simulink model "RefModel_Navfilter"  (R2020b)
settings: Solver=ode1  StartTime=0.0  StopTime=inf  FixedStep=Ts_Navi.Ts_Base  RelTol=1e-3
values from neighbouring files (symbols this model uses):
  NAVI_PARAM_V10 = INIT_Navi_V10(NaviSimParam.Ts_Base)    [SetAlgoParam_Navi.m]
  NAVI_PARAM_V1000 = INIT_Navi_V1000(NaviSimParam.Ts_Base)    [SetAlgoParam_Navi.m]
undefined symbols (not defined in the file or in its folder): ENUM_SensorHealthStatus, NAVI_PARAM_BASE
libraries: aerolibobsolete x1
(part 1 of 2)
settings Model: PauseTimes=[308,310,12]  Creator=sl  LastModifiedBy=sl
settings DataIOCC: SaveOutput=off  SaveTime=off
settings OptimizationCC: DefaultParameterBehavior=Inlined  EnhancedBackFolding=on  PassReuseOutputArgsAs=Individual arguments  ZeroExternalMemoryAtStartup=off  ZeroInternalMemoryAtStartup=off  OptimizeBlockOrder=speed  DifferentSizesBufferReuse=on  OptimizationCustomize=off  EfficientTunableParamExpr=on
settings DebuggingCC: InheritedTsInSrcMsg=none  ParameterPrecisionLossMsg=none  ParameterTunabilityLossMsg=error  UnconnectedInputMsg=none  UnconnectedOutputMsg=none  UnconnectedLineMsg=none  SFUnusedDataAndEventsDiag=none
settings HardwareCC: ProdBitPerPointer=32  ProdBitPerSizeT=32  ProdBitPerPtrDiffT=32  ProdLargestAtomicInteger=Long  ProdLargestAtomicFloat=Double  ProdWordSize=32  ProdHWDeviceType=ARM Compatible->ARM Cortex
settings ModelReferenceCC: ModelReferenceNumInstancesAllowed=Single
settings SFSimCC: MATLABDynamicMemAlloc=off
settings RTWCC: Description=Embedded Coder  SystemTargetFile=ert.tlc  TemplateMakefile=ert_default_tmf  GenerateReport=on  IncludeHyperlinkInReport=on  LaunchReport=on  GenerateTraceInfo=on  GenerateTraceReport=on  GenerateTraceReportSl=on  GenerateTraceReportSf=on  GenerateTraceReportEml=on
settings CodeAppCC: ForceParamTrailComments=on  IgnoreCustomStorageClasses=off  MaxIdLength=48  OperatorAnnotations=on  SimulinkDataObjDesc=on  SFDataObjDesc=on  InsertBlockDesc=on
settings ERTTargetCC: TargetLangStandard=C99 (ISO)  GenerateSampleERTMain=on  CombineOutputUpdateFcns=off  LogVarNameModifier=none  SupportVariableSizeSignals=on  InlinedParameterPlacement=NonHierarchical  ERTCustomFileTemplate=example_file_process.tlc

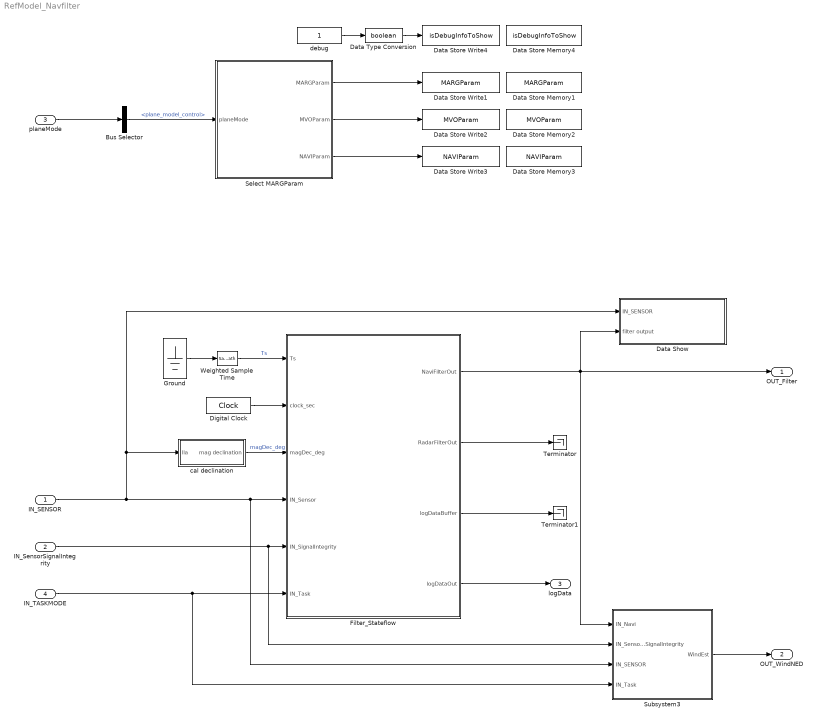
== system RefModel_Navfilter ==
  IN_SENSOR : Inport  OutDataTypeStr=Bus: BUS_SENSOR  BusOutputAsStruct=on
  IN_SensorSignalIntegrity : Inport  Port=2  OutDataTypeStr=Bus: BUS_NAVI_SensorSignalIntegrity  BusOutputAsStruct=on
  planeMode : Inport  Port=3  OutDataTypeStr=Bus: BUS_SYSTEMINFO_INPUT
  IN_TASKMODE : Inport  Port=4  OutDataTypeStr=Bus: BUS_TASK_PATH_OutParam  BusOutputAsStruct=on
  Bus Selector : BusSelector  OutputSignals=plane_model_control
  Data Show : Subsystem
  Data Store Memory1 : DataStoreMemory  DataStoreName=MARGParam  ReadBeforeWriteMsg=warning  WriteAfterWriteMsg=warning  WriteAfterReadMsg=warning  ShowAdditionalParam=off  OutDataTypeStr=Bus: BUS_NAVIPARAM_MARG  Dimensions=1
  Data Store Memory2 : DataStoreMemory  DataStoreName=MVOParam  ReadBeforeWriteMsg=warning  WriteAfterWriteMsg=warning  WriteAfterReadMsg=warning  ShowAdditionalParam=off  OutDataTypeStr=Bus: BUS_NAVIPARAM_MVO  Dimensions=1
  Data Store Memory3 : DataStoreMemory  DataStoreName=NAVIParam  ReadBeforeWriteMsg=warning  WriteAfterWriteMsg=warning  WriteAfterReadMsg=warning  ShowAdditionalParam=off  OutDataTypeStr=Bus: BUS_NAVIPARAM  Dimensions=1
  Data Store Memory4 : DataStoreMemory  DataStoreName=isDebugInfoToShow  ReadBeforeWriteMsg=warning  WriteAfterWriteMsg=warning  WriteAfterReadMsg=warning  ShowAdditionalParam=off  OutDataTypeStr=boolean  Dimensions=1
  Data Store Write1 : DataStoreWrite  DataStoreName=MARGParam
  Data Store Write2 : DataStoreWrite  DataStoreName=MVOParam
  Data Store Write3 : DataStoreWrite  DataStoreName=NAVIParam
  Data Store Write4 : DataStoreWrite  DataStoreName=isDebugInfoToShow
  Data Type Conversion : DataTypeConversion  OutDataTypeStr=boolean
  Digital Clock : DigitalClock  SampleTime=-1
  Filter_Stateflow : Stateflow chart  TreatAsAtomicUnit=on
      settings: PortSchema="{\"entries\":[{\"content\":{\"sides\":[{\"content\":{\"connectorIds\":[\"In1\",\"In2\",\"In3\",\"In4\",\"In5\",\"In6\"]},\"type\":\"ConnectorPlacement.EquallySpacedRectSide\",\"uuid\":\"09dead05-b0d6-46e3-b4df-7e330e053911\"},{\"content\":{\"connectorIds\":[\"Out2\",\"Out1\",\"Out3\",\"Out4\"],\"side\":\"RIGHT\"},\"type\":\"ConnectorPlacement.EquallySpacedRectSide\",\"uuid\":\"42007dbc-3269-4462-8f8b-2c35f13a3107\"},{\"content\":{\"connectorIds\":[],\"side\":\"TOP\"},\"type\":\"ConnectorPlacement.EquallySpacedRectSide\",\"uuid\":\"e6ce5443-da4b-4773-901c-23b39c5492a3\"}]},\"type\":\"ConnectorPlacement.EquallySpacedConnector\",\"uuid\":\"f5fda4a3-ef90-4dff-b16b-01a3b267f071\"}],\"packageUris\":[\"http://schema.mathworks.com/mf0/Connector/R2020b\"],\"version\":\"1.0\"}"
  Ground : Ground
  Select MARGParam : Subsystem
  Subsystem3 : Subsystem
  Terminator : Terminator
  Terminator1 : Terminator
  Weighted Sample Time : SampleTimeMath  TsampMathOp=Ts Only
  cal declination : Subsystem
  debug : Constant
  OUT_Filter : Outport  OutDataTypeStr=Bus: BUS_NAVI_FilterOut  BusOutputAsStruct=on
  OUT_WindNED : Outport  Port=2  OutDataTypeStr=Bus: BUS_NAVI_GlobalWindEst  BusOutputAsStruct=on
  logData : Outport  Port=3  OutDataTypeStr=Bus: BUS_NAVI_SingleLog  BusOutputAsStruct=on
  wires:
  IN_SensorSignalIntegrity/1 -> Subsystem3/2(IN_SensorSignalIntegrity), Filter_Stateflow/5(IN_SignalIntegrity)
  IN_SENSOR/1 -> cal declination/1(lla), Data Show/1(IN_SENSOR), Subsystem3/3(IN_SENSOR), Filter_Stateflow/4(IN_Sensor)
  Digital Clock/1 -> Filter_Stateflow/2(clock_sec)
  Weighted Sample Time/1 -> Filter_Stateflow/1(Ts)  "Ts"
  Ground/1 -> Weighted Sample Time/1
  Subsystem3/1(WindEst) -> OUT_WindNED/1
  Select MARGParam/1(MARGParam) -> Data Store Write1/1
  planeMode/1 -> Bus Selector/1
  Bus Selector/1 -> Select MARGParam/1(planeMode)  "<plane_model_control>"
  Select MARGParam/2(MVOParam) -> Data Store Write2/1
  Select MARGParam/3(NAVIParam) -> Data Store Write3/1
  IN_TASKMODE/1 -> Subsystem3/4(IN_Task), Filter_Stateflow/6(IN_Task)
  cal declination/1(mag declination) -> Filter_Stateflow/3(magDec_deg)  "magDec_deg"
  Data Type Conversion/1 -> Data Store Write4/1
  debug/1 -> Data Type Conversion/1
  Filter_Stateflow/4(logDataOut) -> logData/1
  Filter_Stateflow/2(NaviFilterOut) -> Subsystem3/1(IN_Navi), OUT_Filter/1, Data Show/2(filter output)
  Filter_Stateflow/1(RadarFilterOut) -> Terminator/1
  Filter_Stateflow/3(logDataBuffer) -> Terminator1/1

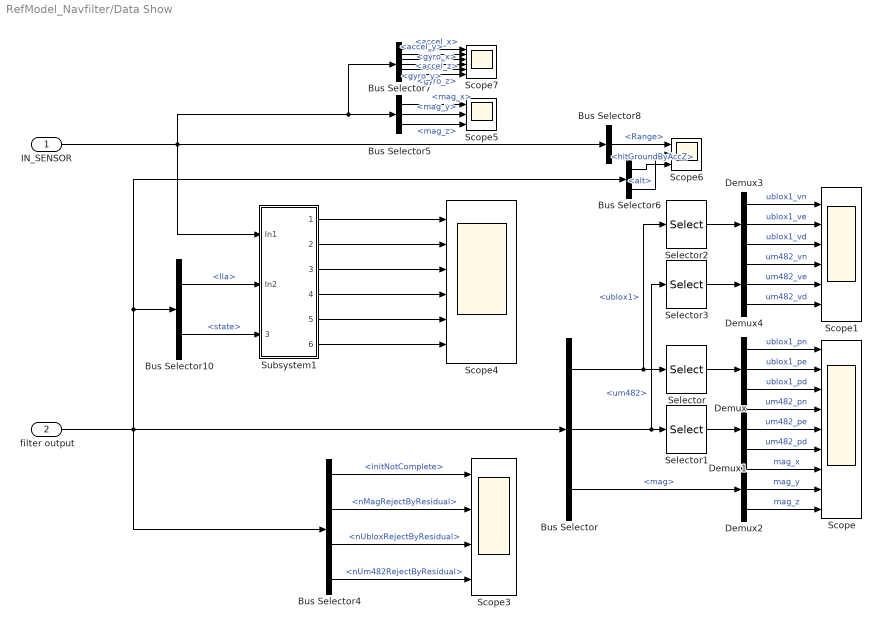
== system RefModel_Navfilter/Data Show ==
  IN_SENSOR : Inport
  filter output : Inport  Port=2
  Bus Selector : BusSelector  OutputSignals=innovMARG.ublox1,innovMARG.um482,innovMARG.mag
  Bus Selector10 : BusSelector  OutputSignals=lla,state
  Bus Selector4 : BusSelector  OutputSignals=Status.initNotComplete,Status.nMagRejectByResidual,Status.nUbloxRejectByResidual,Status.nUm482RejectByResidual
  Bus Selector5 : BusSelector  OutputSignals=mag2.mag_x,mag2.mag_y,mag2.mag_z
  Bus Selector6 : BusSelector  OutputSignals=hitGroundByAccZ,alt
  Bus Selector7 : BusSelector  OutputSignals=IMU1.accel_x,IMU1.accel_y,IMU1.accel_z,IMU1.gyro_x,IMU1.gyro_y,IMU1.gyro_z
  Bus Selector8 : BusSelector  OutputSignals=radar1.Range
  Demux{,1..4} (5 alike) : Demux  Outputs=3
  Scope : Scope  NumInputPorts=9
  Scope1 : Scope  NumInputPorts=6
  Scope3 : Scope  NumInputPorts=4
  Scope4 : Scope  NumInputPorts=6
  Scope5 : Scope  NumInputPorts=3
  Scope6 : Scope  NumInputPorts=3
  Scope7 : Scope  NumInputPorts=6
  Selector : Selector  InputPortWidth=6  IndexOptions=Index vector (dialog)  Indices=[1:3]  OutputSizes=1
  Selector1 : Selector  InputPortWidth=6  IndexOptions=Index vector (dialog)  Indices=[1:3]  OutputSizes=1
  Selector2 : Selector  InputPortWidth=6  IndexOptions=Index vector (dialog)  Indices=[4:6]  OutputSizes=1
  Selector3 : Selector  InputPortWidth=6  IndexOptions=Index vector (dialog)  Indices=[4:6]  OutputSizes=1
  Subsystem1 : Subsystem
  wires:
  Demux/3 -> Scope/3  "ublox1_pd"
  Subsystem1/5(Out5) -> Scope4/5
  IN_SENSOR/1 -> Subsystem1/1(In1), Bus Selector7/1, Bus Selector5/1, Bus Selector8/1
  Bus Selector10/2 -> Subsystem1/3(stateEst)  "<state>"
  Demux2/1 -> Scope/7  "mag_x"
  Bus Selector10/1 -> Subsystem1/2(In2)  "<lla>"
  Subsystem1/6(Out6) -> Scope4/6
  Demux2/2 -> Scope/8  "mag_y"
  Bus Selector5/3 -> Scope5/3  "<mag_z>"
  Demux1/1 -> Scope/4  "um482_pn"
  Selector3/1 -> Demux4/1
  Demux/2 -> Scope/2  "ublox1_pe"
  Demux3/3 -> Scope1/3  "ublox1_vd"
  Bus Selector7/4 -> Scope7/4  "<gyro_x>"
  Bus Selector/2 -> Selector3/1, Selector1/1  "<um482>"
  Bus Selector7/6 -> Scope7/6  "<gyro_z>"
  Bus Selector/1 -> Selector2/1, Selector/1  "<ublox1>"
  Demux1/3 -> Scope/6  "um482_pd"
  Selector/1 -> Demux/1
  Bus Selector7/5 -> Scope7/5  "<gyro_y>"
  Bus Selector5/1 -> Scope5/1  "<mag_x>"
  Demux4/1 -> Scope1/4  "um482_vn"
  Demux4/2 -> Scope1/5  "um482_ve"
  Demux/1 -> Scope/1  "ublox1_pn"
  Bus Selector7/1 -> Scope7/1  "<accel_x>"
  Bus Selector/3 -> Demux2/1  "<mag>"
  Demux4/3 -> Scope1/6  "um482_vd"
  Demux3/2 -> Scope1/2  "ublox1_ve"
  Selector2/1 -> Demux3/1
  Bus Selector7/3 -> Scope7/3  "<accel_z>"
  Subsystem1/4(Out4) -> Scope4/4
  Demux1/2 -> Scope/5  "um482_pe"
  Subsystem1/1(Out1) -> Scope4/1
  Demux3/1 -> Scope1/1  "ublox1_vn"
  Demux2/3 -> Scope/9  "mag_z"
  Bus Selector5/2 -> Scope5/2  "<mag_y>"
  Subsystem1/2(Out2) -> Scope4/2
  Bus Selector6/1 -> Scope6/3  "<hitGroundByAccZ>"
  Bus Selector7/2 -> Scope7/2  "<accel_y>"
  Bus Selector6/2 -> Scope6/2  "<alt>"
  Subsystem1/3(Out3) -> Scope4/3
  Bus Selector8/1 -> Scope6/1  "<Range>"
  Selector1/1 -> Demux1/1
  Bus Selector4/2 -> Scope3/2  "<nMagRejectByResidual>"
  Bus Selector4/1 -> Scope3/1  "<initNotComplete>"
  Bus Selector4/4 -> Scope3/4  "<nUm482RejectByResidual>"
  Bus Selector4/3 -> Scope3/3  "<nUbloxRejectByResidual>"
  filter output/1 -> Bus Selector4/1, Bus Selector/1, Bus Selector6/1, Bus Selector10/1

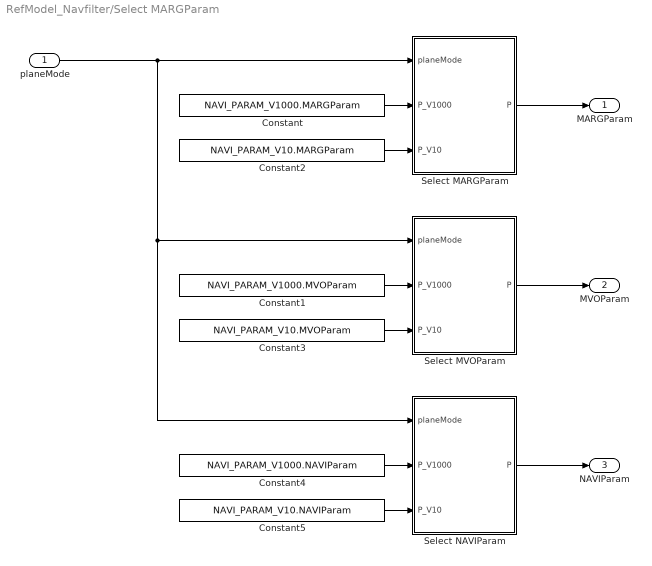
== system RefModel_Navfilter/Select MARGParam ==
  planeMode : Inport
  Constant : Constant  Value=NAVI_PARAM_V1000.MARGParam  OutDataTypeStr=Bus: BUS_NAVIPARAM_MARG
  Constant1 : Constant  Value=NAVI_PARAM_V1000.MVOParam  OutDataTypeStr=Bus: BUS_NAVIPARAM_MVO
  Constant2 : Constant  Value=NAVI_PARAM_V10.MARGParam  OutDataTypeStr=Bus: BUS_NAVIPARAM_MARG
  Constant3 : Constant  Value=NAVI_PARAM_V10.MVOParam  OutDataTypeStr=Bus: BUS_NAVIPARAM_MVO
  Constant4 : Constant  Value=NAVI_PARAM_V1000.NAVIParam  OutDataTypeStr=Bus: BUS_NAVIPARAM
  Constant5 : Constant  Value=NAVI_PARAM_V10.NAVIParam  OutDataTypeStr=Bus: BUS_NAVIPARAM
  Select MARGParam : MATLAB Function  TreatAsAtomicUnit=on
  Select MVOParam : MATLAB Function  TreatAsAtomicUnit=on
  Select NAVIParam : MATLAB Function  TreatAsAtomicUnit=on
  MARGParam : Outport
  MVOParam : Outport  Port=2
  NAVIParam : Outport  Port=3
  wires:
  Constant/1 -> Select MARGParam/2(P_V1000)
  Constant2/1 -> Select MARGParam/3(P_V10)
  Select MARGParam/1(P) -> MARGParam/1
  Select MVOParam/1(P) -> MVOParam/1
  Constant3/1 -> Select MVOParam/3(P_V10)
  Constant1/1 -> Select MVOParam/2(P_V1000)
  Constant4/1 -> Select NAVIParam/2(P_V1000)
  Constant5/1 -> Select NAVIParam/3(P_V10)
  Select NAVIParam/1(P) -> NAVIParam/1
  planeMode/1 -> Select MARGParam/1(planeMode), Select NAVIParam/1(planeMode), Select MVOParam/1(planeMode)

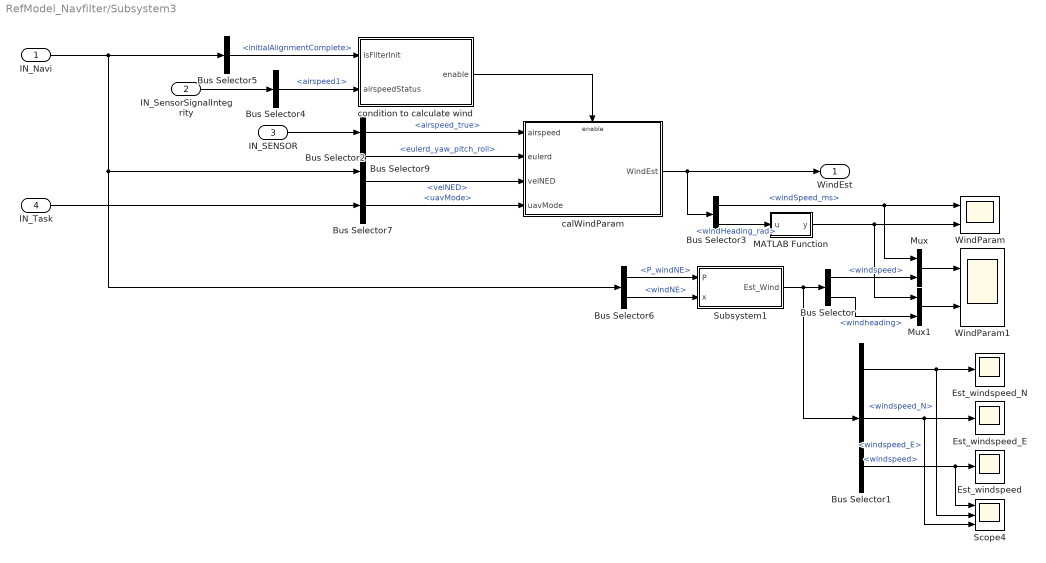
== system RefModel_Navfilter/Subsystem3 ==
  IN_Navi : Inport
  IN_SensorSignalIntegrity : Inport  Port=2
  IN_SENSOR : Inport  Port=3
  IN_Task : Inport  Port=4
  Bus Selector : BusSelector  OutputSignals=windspeed,windheading
  Bus Selector1 : BusSelector  OutputSignals=windspeed_N,windspeed_E,windspeed
  Bus Selector2 : BusSelector  OutputSignals=airspeed1.airspeed_true
  Bus Selector3 : BusSelector  OutputSignals=windSpeed_ms,windHeading_rad
  Bus Selector4 : BusSelector  OutputSignals=SensorStatus.airspeed1
  Bus Selector5 : BusSelector  OutputSignals=Status.initialAlignmentComplete
  Bus Selector6 : BusSelector  OutputSignals=Covariance.P_windNE,windNE
  Bus Selector7 : BusSelector  OutputSignals=uavMode
  Bus Selector9 : BusSelector  OutputSignals=eulerd_yaw_pitch_roll,velNED
  Est_windspeed : Scope
  Est_windspeed_E : Scope
  Est_windspeed_N : Scope
  MATLAB Function : MATLAB Function  TreatAsAtomicUnit=on
  Mux : Mux  Inputs=2
  Mux1 : Mux  Inputs=2
  Scope4 : Scope  NumInputPorts=3
  Subsystem1 : Subsystem
  WindParam : Scope  NumInputPorts=2
  WindParam1 : Scope  NumInputPorts=2
  calWindParam : Subsystem
  condition to calculate wind : Subsystem
  WindEst : Outport
  wires:
  Bus Selector9/2 -> calWindParam/3(velNED)  "<velNED>"
  IN_SENSOR/1 -> Bus Selector2/1
  calWindParam/1(WindEst) -> WindEst/1, Bus Selector3/1
  Bus Selector3/1 -> Mux/1, WindParam/1  "<windSpeed_ms>"
  Bus Selector3/2 -> MATLAB Function/1(u)  "<windHeading_rad>"
  IN_Navi/1 -> Bus Selector5/1, Bus Selector9/1, Bus Selector6/1
  Bus Selector9/1 -> calWindParam/2(eulerd)  "<eulerd_yaw_pitch_roll>"
  Bus Selector2/1 -> calWindParam/1(airspeed)  "<airspeed_true>"
  Subsystem1/1(Est_Wind) -> Bus Selector1/1, Bus Selector/1
  Mux/1 -> WindParam1/1
  Mux1/1 -> WindParam1/2
  Bus Selector/1 -> Mux/2  "<windspeed>"
  Bus Selector/2 -> Mux1/2  "<windheading>"
  MATLAB Function/1(y) -> Mux1/1, WindParam/2
  IN_Task/1 -> Bus Selector7/1
  Bus Selector1/2 -> Scope4/3, Est_windspeed_E/1  "<windspeed_E>"
  Bus Selector1/3 -> Scope4/1, Est_windspeed/1  "<windspeed>"
  Bus Selector1/1 -> Scope4/2, Est_windspeed_N/1  "<windspeed_N>"
  Bus Selector6/1 -> Subsystem1/1(P)  "<P_windNE>"
  Bus Selector6/2 -> Subsystem1/2(x)  "<windNE>"
  IN_SensorSignalIntegrity/1 -> Bus Selector4/1
  condition to calculate wind/1(enable) -> calWindParam/Enable
  Bus Selector5/1 -> condition to calculate wind/1(isFilterInit)  "<initialAlignmentComplete>"
  Bus Selector4/1 -> condition to calculate wind/2(airspeedStatus)  "<airspeed1>"
  Bus Selector7/1 -> calWindParam/4(uavMode)  "<uavMode>"

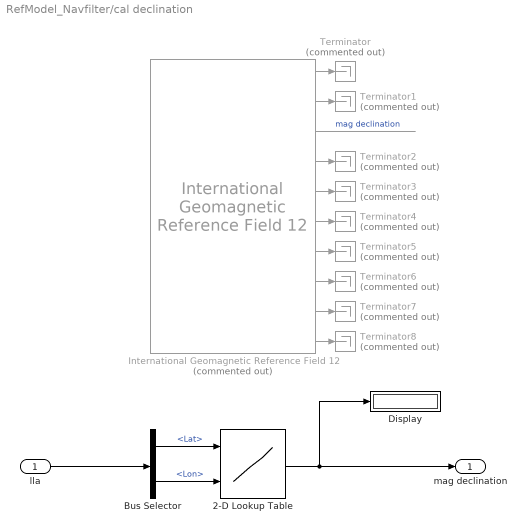
== system RefModel_Navfilter/cal declination ==
  lla : Inport
  2-D Lookup Table : Lookup_n-D  BreakpointsForDimension1=NAVI_PARAM_BASE.magneticData_igrfmagm.lat  BreakpointsForDimension2=NAVI_PARAM_BASE.magneticData_igrfmagm.lon  Table=NAVI_PARAM_BASE.magneticData_igrfmagm.magDec  ExtrapMethod=Clip  UseLastTableValue=on  InternalRulePriority=Speed  RndMeth=Simplest  InputSameDT=on
      settings: InputPortMap=u0,u1
  Bus Selector : BusSelector  OutputSignals=ublox1.Lat,ublox1.Lon
  Display : Display
  International Geomagnetic Reference Field 12 : aerolibobsolete/International Geomagnetic Reference Field 12  Commented=on  units=Metric (MKS)  time_in=off  month=December  day=20  year=2019  action=None  sv_out=on
      settings: SourceProductBaseCode=AE
  Terminator{,1..8} (9 alike) : Terminator  Commented=on
  mag declination : Outport
  wires:
  International Geomagnetic Reference Field 12/9 -> Terminator7/1
  International Geomagnetic Reference Field 12/10 -> Terminator8/1
  International Geomagnetic Reference Field 12/4 -> Terminator2/1
  International Geomagnetic Reference Field 12/1 -> Terminator/1
  International Geomagnetic Reference Field 12/2 -> Terminator1/1
  International Geomagnetic Reference Field 12/3 -> ?  "mag declination"
  International Geomagnetic Reference Field 12/5 -> Terminator3/1
  International Geomagnetic Reference Field 12/6 -> Terminator4/1
  International Geomagnetic Reference Field 12/8 -> Terminator6/1
  International Geomagnetic Reference Field 12/7 -> Terminator5/1
  lla/1 -> Bus Selector/1
  2-D Lookup Table/1 -> mag declination/1, Display/1
  Bus Selector/1 -> 2-D Lookup Table/1  "<Lat>"
  Bus Selector/2 -> 2-D Lookup Table/2  "<Lon>"

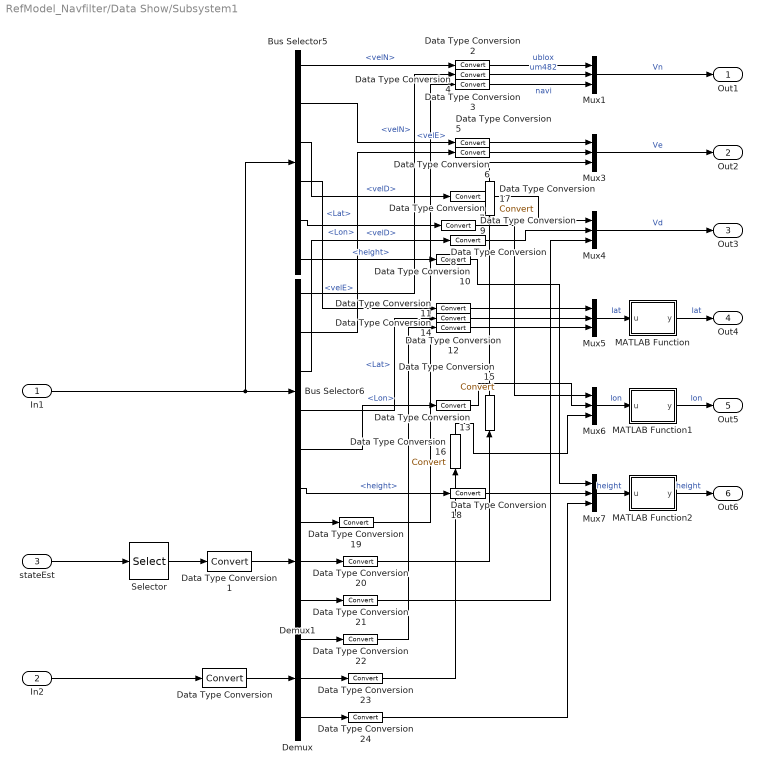
== system RefModel_Navfilter/Data Show/Subsystem1 ==
  In1 : Inport
  In2 : Inport  Port=2
  stateEst : Inport  Port=3
  Bus Selector5 : BusSelector  OutputSignals=ublox1.velN,ublox1.velE,ublox1.velD,ublox1.Lat,ublox1.Lon,ublox1.height
  Bus Selector6 : BusSelector  OutputSignals=um482.velN,um482.velE,um482.velD,um482.Lat,um482.Lon,um482.height
  Data Type Conversion{,1..24} (25 alike) : DataTypeConversion
  Demux : Demux  Outputs=3
  Demux1 : Demux  Outputs=3
  MATLAB Function : MATLAB Function  TreatAsAtomicUnit=on
  MATLAB Function1 : MATLAB Function  TreatAsAtomicUnit=on
  MATLAB Function2 : MATLAB Function  TreatAsAtomicUnit=on
  Mux{1,3..7} (6 alike) : Mux  Inputs=3
  Selector : Selector  InputPortWidth=24  IndexOptions=Index vector (dialog)  Indices=[8 9 10]  OutputSizes=1
  Out1 : Outport
  Out2 : Outport  Port=2
  Out3 : Outport  Port=3
  Out4 : Outport  Port=4
  Out5 : Outport  Port=5
  Out6 : Outport  Port=6
  wires:
  Bus Selector5/3 -> Data Type Conversion7/1  "<velD>"
  Mux3/1 -> Out2/1  "Ve"
  Demux/3 -> Data Type Conversion24/1
  Demux/2 -> Data Type Conversion23/1
  Bus Selector5/4 -> Data Type Conversion11/1  "<Lat>"
  Demux/1 -> Data Type Conversion22/1
  Demux1/3 -> Data Type Conversion21/1
  Bus Selector5/6 -> Data Type Conversion10/1  "<height>"
  Bus Selector6/1 -> Data Type Conversion3/1  "<velN>"
  Bus Selector6/3 -> Data Type Conversion8/1  "<velD>"
  Bus Selector6/6 -> Data Type Conversion18/1  "<height>"
  Bus Selector6/4 -> Data Type Conversion12/1  "<Lat>"
  Mux5/1 -> MATLAB Function/1(u)  "lat"
  Bus Selector5/2 -> Data Type Conversion5/1  "<velE>"
  Demux1/1 -> Data Type Conversion19/1
  Bus Selector6/2 -> Data Type Conversion6/1  "<velE>"
  Bus Selector6/5 -> Data Type Conversion13/1  "<Lon>"
  Bus Selector5/1 -> Data Type Conversion2/1  "<velN>"
  Bus Selector5/5 -> Data Type Conversion9/1  "<Lon>"
  Mux1/1 -> Out1/1  "Vn"
  Demux1/2 -> Data Type Conversion20/1
  In2/1 -> Data Type Conversion/1
  Mux4/1 -> Out3/1  "Vd"
  Mux7/1 -> MATLAB Function2/1(u)  "height"
  Mux6/1 -> MATLAB Function1/1(u)  "lon"
  stateEst/1 -> Selector/1
  Selector/1 -> Data Type Conversion1/1
  Data Type Conversion/1 -> Demux/1
  Data Type Conversion1/1 -> Demux1/1
  In1/1 -> Bus Selector5/1, Bus Selector6/1
  Data Type Conversion2/1 -> Mux1/1  "ublox"
  Data Type Conversion3/1 -> Mux1/2  "um482"
  Data Type Conversion4/1 -> Mux1/3  "navi"
  Data Type Conversion5/1 -> Mux3/1
  Data Type Conversion6/1 -> Mux3/2
  Data Type Conversion7/1 -> Mux4/1
  Data Type Conversion8/1 -> Mux4/2
  Data Type Conversion9/1 -> Mux6/1
  Data Type Conversion10/1 -> Mux7/1
  Data Type Conversion11/1 -> Mux5/1
  Data Type Conversion12/1 -> Mux5/2
  Data Type Conversion14/1 -> Mux5/3
  Data Type Conversion13/1 -> Mux6/2
  Data Type Conversion15/1 -> Data Type Conversion17/1
  Data Type Conversion16/1 -> Mux6/3
  Data Type Conversion17/1 -> Mux3/3
  Data Type Conversion18/1 -> Mux7/2
  Data Type Conversion19/1 -> Data Type Conversion4/1
  Data Type Conversion20/1 -> Data Type Conversion15/1
  Data Type Conversion21/1 -> Mux4/3
  Data Type Conversion22/1 -> Data Type Conversion14/1
  Data Type Conversion23/1 -> Data Type Conversion16/1
  Data Type Conversion24/1 -> Mux7/3
  MATLAB Function/1(y) -> Out4/1  "lat"
  MATLAB Function1/1(y) -> Out5/1  "lon"
  MATLAB Function2/1(y) -> Out6/1  "height"

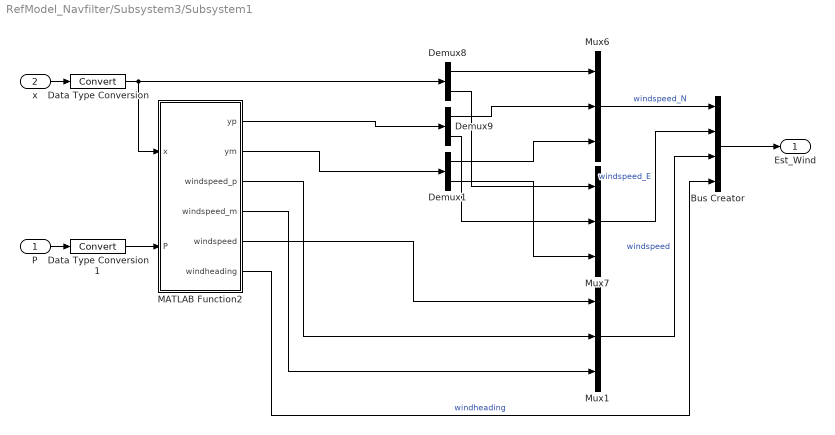
== system RefModel_Navfilter/Subsystem3/Subsystem1 ==
  P : Inport
  x : Inport  Port=2
  Bus Creator : BusCreator  Inputs=4
  Data Type Conversion : DataTypeConversion
  Data Type Conversion1 : DataTypeConversion
  Demux1 : Demux  Outputs=2
  Demux8 : Demux  Outputs=2
  Demux9 : Demux  Outputs=2
  MATLAB Function2 : MATLAB Function  TreatAsAtomicUnit=on
  Mux1 : Mux  Inputs=3
  Mux6 : Mux  Inputs=3
  Mux7 : Mux  Inputs=3
  Est_Wind : Outport
  wires:
  Demux9/1 -> Mux6/2
  Demux8/2 -> Mux7/1
  Demux8/1 -> Mux6/1
  Demux9/2 -> Mux7/2
  Mux6/1 -> Bus Creator/1  "windspeed_N"
  x/1 -> Data Type Conversion/1
  P/1 -> Data Type Conversion1/1
  Mux7/1 -> Bus Creator/2  "windspeed_E"
  MATLAB Function2/6(windheading) -> Bus Creator/4  "windheading"
  Bus Creator/1 -> Est_Wind/1
  Demux1/1 -> Mux6/3
  Demux1/2 -> Mux7/3
  MATLAB Function2/1(yp) -> Demux9/1
  MATLAB Function2/2(ym) -> Demux1/1
  Mux1/1 -> Bus Creator/3  "windspeed"
  Data Type Conversion/1 -> Demux8/1, MATLAB Function2/1(x)
  Data Type Conversion1/1 -> MATLAB Function2/2(P)
  MATLAB Function2/3(windspeed_p) -> Mux1/2
  MATLAB Function2/4(windspeed_m) -> Mux1/3
  MATLAB Function2/5(windspeed) -> Mux1/1

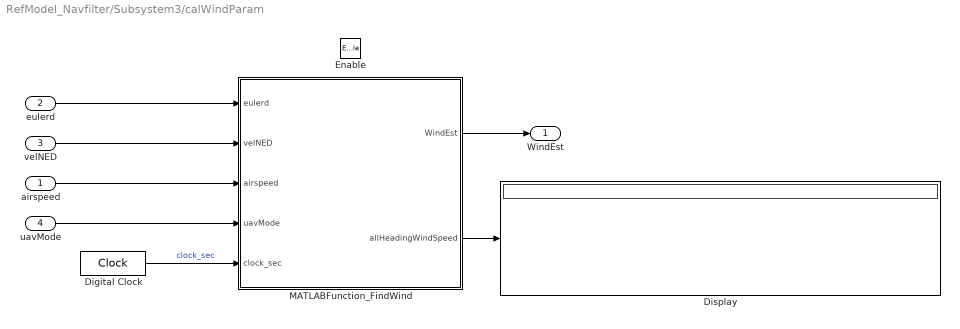
== system RefModel_Navfilter/Subsystem3/calWindParam ==
  airspeed : Inport
  eulerd : Inport  Port=2
  velNED : Inport  Port=3
  uavMode : Inport  Port=4
  Enable : EnablePort
  Digital Clock : DigitalClock  SampleTime=-1
  Display : Display
  MATLABFunction_FindWind : MATLAB Function  TreatAsAtomicUnit=on
  WindEst : Outport
  wires:
  eulerd/1 -> MATLABFunction_FindWind/1(eulerd)
  airspeed/1 -> MATLABFunction_FindWind/3(airspeed)
  MATLABFunction_FindWind/1(WindEst) -> WindEst/1
  MATLABFunction_FindWind/2(allHeadingWindSpeed) -> Display/1
  velNED/1 -> MATLABFunction_FindWind/2(velNED)
  uavMode/1 -> MATLABFunction_FindWind/4(uavMode)
  Digital Clock/1 -> MATLABFunction_FindWind/5(clock_sec)  "clock_sec"

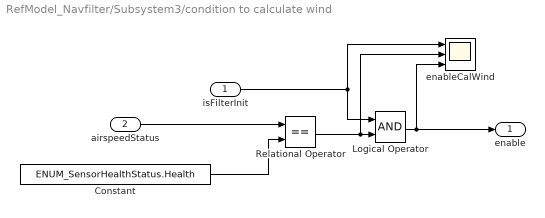
== system RefModel_Navfilter/Subsystem3/condition to calculate wind ==
  isFilterInit : Inport
  airspeedStatus : Inport  Port=2
  Constant : Constant  Value=ENUM_SensorHealthStatus.Health  OutDataTypeStr=Enum: ENUM_SensorHealthStatus
  Logical Operator : Logic  AllPortsSameDT=off  OutDataTypeStr=boolean
  Relational Operator : RelationalOperator  Operator===  OutDataTypeStr=boolean  RndMeth=Simplest
  enableCalWind : Scope  NumInputPorts=3
  enable : Outport
  wires:
  Relational Operator/1 -> enableCalWind/2, Logical Operator/2
  isFilterInit/1 -> enableCalWind/1, Logical Operator/1
  Logical Operator/1 -> enable/1, enableCalWind/3
  airspeedStatus/1 -> Relational Operator/1
  Constant/1 -> Relational Operator/2

== matlab function RefModel_Navfilter/Subsystem3/Subsystem1/MATLAB Function2 ==
  data: yp output; x input; P input; ym output; windspeed_p output; windspeed_m output; windspeed output; windheading output
function [yp,ym,windspeed_p,windspeed_m,windspeed,windheading] = fcn(x, P)
% 3 sigma
yp = x + 3*sqrt(P);
ym = x - 3*sqrt(P);

windspeed = norm(x);
windspeed_p = windspeed + 3*norm(sqrt(P));
windspeed_m = windspeed - 3*norm(sqrt(P));

windheading = atan2(x(1),x(2));

== matlab function RefModel_Navfilter/Subsystem3/calWindParam/MATLABFunction_FindWind ==
  data: eulerd input; velNED input; airspeed input; WindEst output Bus: BUS_NAVI_GlobalWindEst; allHeadingWindSpeed output; uavMode input; clock_sec input
function [WindEst,allHeadingWindSpeed] = findWind(eulerd,velNED, airspeed,uavMode, clock_sec)
persistent gsBuffer heading0_deg oneCircleComplete idxsel airspeed_filter
persistent preWindSpeed_ms
nanflag = -9999;
heading_deg = eulerd(1);
pitch_deg = eulerd(2);
if isempty(gsBuffer)
%     fprintf('Start find wind\n');
    gsBuffer = nanflag*ones(36,1);
    heading0_deg = heading_deg;
    oneCircleComplete = false;
    airspeed_filter = airspeed;
    preWindSpeed_ms = 0;
    idxsel = -1;
end
k_filter = 0.8;
airspeed_filter = k_filter*airspeed_filter + (1-k_filter)*airspeed;
groundSpeed = norm(velNED(1:2));
stepAngle = 360/length(gsBuffer);
curHeading_deg = heading_deg;
velHeading_deg = atan2(velNED(2),velNED(1))*180/pi;
dHeading_deg = angdiff(curHeading_deg*pi/180,velHeading_deg*pi/180)*180/pi;
temp = 70;
if dHeading_deg > temp
    dHeading_deg = temp;
elseif dHeading_deg < -temp
    dHeading_deg = -temp;
end

gpsvel_alongUavHeading = norm(velNED(1:3))*cos(dHeading_deg*pi/180);
vel = airspeed_filter-gpsvel_alongUavHeading; 
% vel = airspeed - norm(velNED(1:3));
diffHeading_deg = angdiff(curHeading_deg*pi/180,heading0_deg*pi/180)*180/pi;
if diffHeading_deg < 0
    diffHeading_deg = diffHeading_deg + 360;
end
if vel < -5
    vel = - vel;
    curHeading_deg = curHeading_deg - 180;
    curHeading_deg = rem(curHeading_deg,360);
    if curHeading_deg > 180
        curHeading_deg = curHeading_deg - 360;
    elseif curHeading_deg < -180
        curHeading_deg = curHeading_deg + 360;
    end
end
if clock_sec > 1300
    sl = 1;
end
% if oneCircleComplete
%     if abs(angdiff((idxsel-1/2)*stepAngle*pi/180,curHeading_deg*pi/180)) <= stepAngle*pi/180 && ...
%             abs(angdiff((idxsel+1/2)*stepAngle*pi/180,curHeading_deg*pi/180)) <= stepAngle*pi/180
%         flag = true;
%     end
% end
Ksmooth = 0.9;
for idx = 1:length(gsBuffer)
    if curHeading_deg < 0
        curHeading_deg = curHeading_deg + 360;
    end
    if curHeading_deg >= (idx-1)*stepAngle && curHeading_deg < idx*stepAngle
        if abs(gsBuffer(idx)) < 20
            gsBuffer(idx) = Ksmooth*gsBuffer(idx) + (1-Ksmooth)*vel;
        else
            gsBuffer(idx) = vel;
        end
    end
end
% 当收集完360度风速后，按需选择风向出航
maxWindSpeed = 0;
idxsel = 0;
if any(gsBuffer~=nanflag)
    [maxWindSpeed,idxsel_temp] = max(gsBuffer);
    idxsel = idxsel_temp(1); % 防止碰巧有多个极值的情况
    if all(gsBuffer~=nanflag)
        oneCircleComplete = true;
    end
end
WindEst.oneCircleComplete = oneCircleComplete;
WindEst.windSpeed_ms = maxWindSpeed; 
WindEst.windHeading_rad = (idxsel+1/2)*stepAngle*pi/180; % 来流方向的反方向
allHeadingWindSpeed = gsBuffer;
if uavMode == ENUM_UAVMode.Rotor || ...
        airspeed_filter <= 10
    if abs(pitch_deg) < 50
        WindEst.windSpeed_ms = double(vel);
    else
        WindEst.windSpeed_ms = preWindSpeed_ms; 
    end
    WindEst.windHeading_rad = double(curHeading_deg)*pi/180;
    preWindSpeed_ms = WindEst.windSpeed_ms;
end
%% 子函数

== matlab function RefModel_Navfilter/Data Show/Subsystem1/MATLAB Function ==
  data: u input; y output
function y = fcn(u)
for i = 1:3
    if u(i) == 0
        u(i) = nan;
    end
end
y = u;

== matlab function RefModel_Navfilter/Data Show/Subsystem1/MATLAB Function1 ==
  data: u input; y output
function y = fcn(u)
for i = 1:3
    if u(i) == 0
        u(i) = nan;
    end
end
y = u;

== matlab function RefModel_Navfilter/Data Show/Subsystem1/MATLAB Function2 ==
  data: u input; y output
function y = fcn(u)
for i = 1:3
    if u(i) == 0
        u(i) = nan;
    end
end
y = u;

== matlab function RefModel_Navfilter/Select MARGParam/Select MARGParam ==
  data: planeMode input Enum: ENUM_plane_mode; P output Bus: BUS_NAVIPARAM_MARG; P_V1000 input Bus: BUS_NAVIPARAM_MARG; P_V10 input Bus: BUS_NAVIPARAM_MARG
function P = fcn(planeMode,P_V1000,P_V10)
switch planeMode
    case ENUM_plane_mode.V10
        P = P_V10;
    case {ENUM_plane_mode.V1000,ENUM_plane_mode.V10s}
        P = P_V1000;
    otherwise
        P = P_V1000;
end

== matlab function RefModel_Navfilter/Select MARGParam/Select MVOParam ==
  data: planeMode input Enum: ENUM_plane_mode; P output Bus: BUS_NAVIPARAM_MVO; P_V1000 input Bus: BUS_NAVIPARAM_MVO; P_V10 input Bus: BUS_NAVIPARAM_MVO
function P = fcn(planeMode,P_V1000,P_V10)
switch planeMode
    case ENUM_plane_mode.V10
        P = P_V10;
    case {ENUM_plane_mode.V1000,ENUM_plane_mode.V10s}
        P = P_V1000;
    otherwise
        P = P_V1000;
end

== matlab function RefModel_Navfilter/Subsystem3/MATLAB Function ==
  data: u input; y output
function y = fcn(u)
% u = u + pi;
u = rem(u,2*pi);
if u > pi
    u = u - 2*pi;
elseif u < -pi
    u = u + 2*pi;
end
y = u;

== matlab function RefModel_Navfilter/Select MARGParam/Select NAVIParam ==
  data: planeMode input Enum: ENUM_plane_mode; P output Bus: BUS_NAVIPARAM; P_V1000 input Bus: BUS_NAVIPARAM; P_V10 input Bus: BUS_NAVIPARAM
function P = fcn(planeMode,P_V1000,P_V10)
switch planeMode
    case ENUM_plane_mode.V10
        P = P_V10;
    case {ENUM_plane_mode.V1000,ENUM_plane_mode.V10s}
        P = P_V1000;
    otherwise
        P = P_V1000;
end
